simulink model "Uebung11_simulink"  (Simulink 8.1)
settings: Solver=ode23  StartTime=0.0  StopTime=15  MaxStep=1e-2  RelTol=1e-3
values from neighbouring files (symbols this model uses):
  KD = 0.125*Tkrit*KP    (= 1.0314)    [Uebung11.m]
  KI = 2/Tkrit*KP    (= 4.52356020942)    [Uebung11.m]
  KP = 0.6*Kkrit    (= 4.32)    [Uebung11.m]
  T1 = 0.001    [Uebung11.m]
settings Model: Creator=Uli  LastModifiedBy=Uli
settings OptimizationCC: InitFltsAndDblsToZero=on
settings DebuggingCC: SaveWithParameterizedLinksMsg=none  SignalResolutionControl=TryResolveAllWithWarning  MultiTaskDSMMsg=warning  MultiTaskCondExecSysMsg=none  StrictBusMsg=Warning
settings RTWCC: IncludeERTFirstTime=on
settings GRTTargetCC: TargetFcnLib=ansi_tfl_tmw.mat

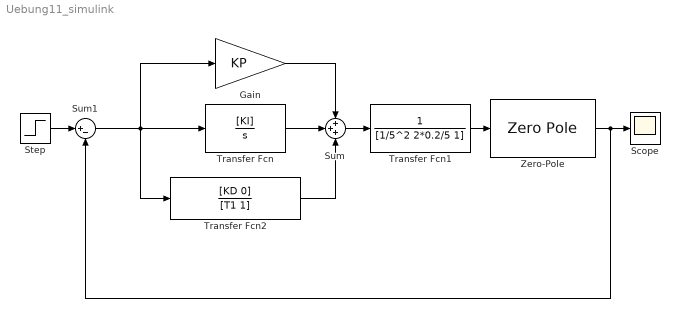
== system Uebung11_simulink ==
  Gain : Gain  Gain=KP
  Scope : Scope
  Step : Step  Time=0  SampleTime=0
  Sum : Sum  Inputs=+++
  Sum1 : Sum  Inputs=|+-
  Transfer Fcn : TransferFcn  Numerator=[KI]  Denominator=[1 0]
  Transfer Fcn1 : TransferFcn  Denominator=[1/5^2 2*0.2/5 1]
  Transfer Fcn2 : TransferFcn  Numerator=[KD 0]  Denominator=[T1 1]
  Zero-Pole : ZeroPole  Zeros=[]  Poles=[ -1 -0.5]
  wires:
  Transfer Fcn/1 -> Sum/2
  Sum1/1 -> Transfer Fcn/1, Transfer Fcn2/1, Gain/1
  Zero-Pole/1 -> Sum1/2, Scope/1
  Step/1 -> Sum1/1
  Sum/1 -> Transfer Fcn1/1
  Transfer Fcn1/1 -> Zero-Pole/1
  Gain/1 -> Sum/1
  Transfer Fcn2/1 -> Sum/3
